simulink subsystem "NoAxleCompliances"  (R2023a)
settings: Solver=VariableStepAuto  StartTime=0.0  StopTime=10.0  RelTol=1e-3
settings Model: Creator=The MathWorks, Inc.  LastModifiedBy=The MathWorks, Inc.

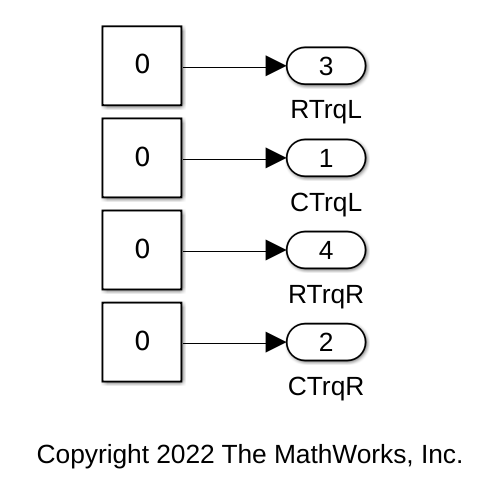
[thumbnail: Simulink's stored preview of the top-level diagram]
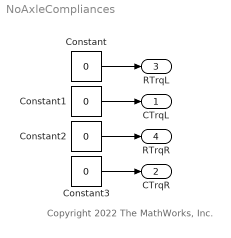
== system NoAxleCompliances ==
  note: Copyright 2022 The MathWorks, Inc.
  Constant{,1..3} (4 alike) : Constant  Value=0  SampleTime=-1
  CTrqL : Outport
  CTrqR : Outport  Port=2
  RTrqL : Outport  Port=3
  RTrqR : Outport  Port=4
  wires:
  Constant2/1 -> RTrqR/1
  Constant1/1 -> CTrqL/1
  Constant/1 -> RTrqL/1
  Constant3/1 -> CTrqR/1
